simulink model "MultiRateCont"  (R2018b)
settings: Solver=ode4  StartTime=0.0  StopTime=10.0  FixedStep=.001  RelTol=1e-3
PreLoadFcn:
  | load 'test_data.mat'
values from neighbouring files (symbols this model uses):
  B = 234    [test_data.mat]
  B_inline = 3.14    [test_data.mat]
  C = 123    [test_data.mat]
libraries: simulink x1
settings Model: SimulationMode=rapid-accelerator  Creator=mmcbroom  LastModifiedBy=slentine
settings DataIOCC: LimitDataPoints=on  SignalLoggingSaveFormat=ModelDataLogs  SaveOutput=off  SignalLogging=off  DSMLogging=off  SaveTime=off
settings OptimizationCC: DefaultParameterBehavior=Inlined  EnhancedBackFolding=on  PassReuseOutputArgsAs=Individual arguments  ExpressionDepthLimit=2147483647  InitFltsAndDblsToZero=on  OptimizeBlockOrder=speed  DifferentSizesBufferReuse=on  OptimizationCustomize=off
settings DebuggingCC: SaveWithParameterizedLinksMsg=none  UnderspecifiedInitializationDetection=Classic  MergeDetectMultiDrivingBlocksExec=none  SolverPrmCheckMsg=warning  ParameterTunabilityLossMsg=error  FcnCallInpInsideContextMsg=warning  BusObjectLabelMismatch=none  StateNameClashWarn=warning  SFUnexpectedBacktrackingDiag=warning  SFNoUnconditionalDefaultTransitionDiag=warning  SFExecutionAtInitializationDiag=none
settings HardwareCC: ProdBitPerPointer=32  ProdBitPerSizeT=32  ProdBitPerPtrDiffT=32  ProdWordSize=32  ProdHWDeviceType=Intel->x86-32 (Windows32)
settings ModelReferenceCC: PropagateSignalLabelsOutOfModel=off
settings SFSimCC: SimUseLocalCustomCode=off  SimParseCustomCode=off  MATLABDynamicMemAlloc=off
settings RTWCC: SystemTargetFile=cfs_ert.tlc  TemplateMakefile=ert_default_tmf  Description=NASA CFS Target File  GenerateReport=on  RTWUseLocalCustomCode=off  IncludeHyperlinkInReport=on  LaunchReport=on  PortableWordSizes=on  GenerateTraceInfo=on  GenerateTraceReport=on  GenerateTraceReportSl=on  GenerateTraceReportSf=on  GenerateTraceReportEml=on
settings CodeAppCC: ForceParamTrailComments=on  IgnoreCustomStorageClasses=off  OperatorAnnotations=on  SimulinkDataObjDesc=on  SFDataObjDesc=on  CustomSymbolStrType=$N$R$M  CustomCommentsFcn=trick_comments.m  InsertBlockDesc=on  EnableCustomComments=on  InternalIdentifier=Classic
settings STFCustomTargetCC: MultiwordLength=256  GenerateSampleERTMain=on  CombineOutputUpdateFcns=on  ERTCustomFileBanners=on  MultiInstanceERTCode=on  CodeInterfacePackaging=Reusable function  SupportNonInlinedSFcns=off  RemoveResetFunc=on  MATLABClassNameForMDSCustomization=Simulink.SoftwareTarget.ERTCustomization  UseToolchainInfoCompliant=on  SystemTargetFile=cfs_ert.tlc
settings ERTTargetCC: GenerateSampleERTMain=on  ParMdlRefBuildCompliant=off  CompOptLevelCompliant=off  ConcurrentExecutionCompliant=off  MultiInstanceERTCode=on  CodeInterfacePackaging=Reusable function  SupportContinuousTime=on  ModelStepFunctionPrototypeControlCompliant=off  CPPClassGenCompliant=off  InlinedParameterPlacement=NonHierarchical  ERTCustomFileTemplate=cfs_interface.tlc
settings ConfigComp: CovMetricSettings=dw  CovHtmlReporting=on  CovSaveCumulativeToWorkspaceVar=on  CovSaveSingleToWorkspaceVar=on  CovExternalEMLEnable=off  CovSFcnEnable=off

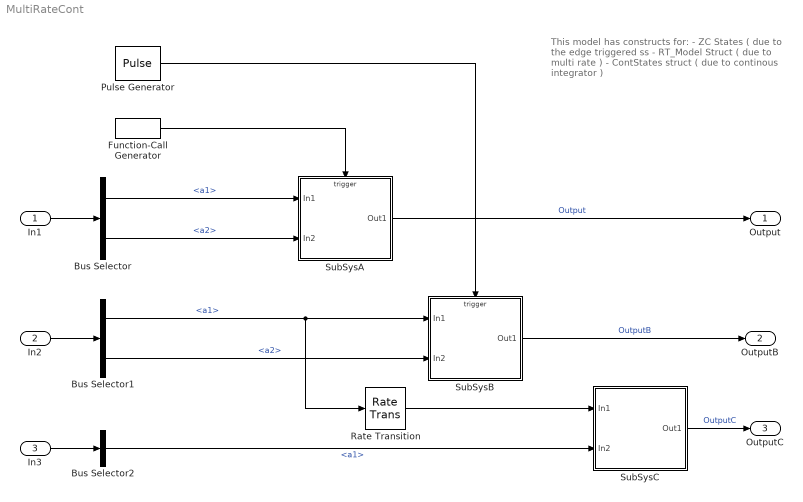
== system MultiRateCont ==
  note: This model has constructs for:
      | - ZC States ( due to the edge triggered ss
      | - RT_Model Struct ( due to multi rate )
      | - ContStates struct ( due to continous integrator )
  In1 : Inport  OutDataTypeStr=Bus: InBus_msg  BusOutputAsStruct=on
  In2 : Inport  Port=2  OutDataTypeStr=Bus: env_cmd_msg  BusOutputAsStruct=on
  In3 : Inport  Port=3  OutDataTypeStr=Bus: InBus_msg  SampleTime=.1  BusOutputAsStruct=on
  Bus Selector : BusSelector  OutputSignals=a1,a2
  Bus Selector1 : BusSelector  OutputSignals=a1,a2
  Bus Selector2 : BusSelector  OutputSignals=a1
  Function-Call Generator : simulink/Ports & Subsystems/Function-Call Generator  sample_time=1  numberOfIterations=1
  Pulse Generator : DiscretePulseGenerator  PulseType=Time based  PulseWidth=50
  Rate Transition : RateTransition  OutPortSampleTime=.1
  SubSysA : Subsystem
      settings: RTWFcnNameOpts=Use subsystem name
  SubSysB : Subsystem
      settings: RTWFcnNameOpts=Use subsystem name
  SubSysC : Subsystem
      settings: RTWSystemCode=Nonreusable function  RTWFcnNameOpts=Use subsystem name  RTWFileNameOpts=Use subsystem name
  Output : Outport
  OutputB : Outport  Port=2
  OutputC : Outport  Port=3
  wires:
  SubSysA/1(Out1) -> Output/1  "Output"
  SubSysB/1(Out1) -> OutputB/1  "OutputB"
  SubSysC/1(Out1) -> OutputC/1  "OutputC"
  Pulse Generator/1 -> SubSysB/Trigger
  Function-Call Generator/1 -> SubSysA/Trigger
  Rate Transition/1 -> SubSysC/1(In1)
  In1/1 -> Bus Selector/1
  Bus Selector/1 -> SubSysA/1(In1)  "<a1>"
  Bus Selector/2 -> SubSysA/2(In2)  "<a2>"
  In2/1 -> Bus Selector1/1
  Bus Selector1/1 -> SubSysB/1(In1), Rate Transition/1  "<a1>"
  Bus Selector1/2 -> SubSysB/2(In2)  "<a2>"
  In3/1 -> Bus Selector2/1
  Bus Selector2/1 -> SubSysC/2(In2)  "<a1>"

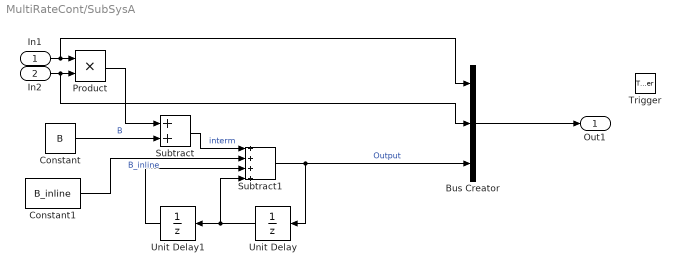
== system MultiRateCont/SubSysA ==
  In1 : Inport
  In2 : Inport  Port=2
  Trigger : TriggerPort  TriggerType=function-call  VariantControl=(inherit)
  Bus Creator : BusCreator  Inputs=3  OutDataTypeStr=Bus: OutBus_msg  NonVirtualBus=on
  Constant : Constant  Value=B
  Constant1 : Constant  Value=B_inline
  Product : Product  RndMeth=Zero
  Subtract : Sum
  Subtract1 : Sum  Inputs=++++
  Unit Delay : UnitDelay  SampleTime=-1  StateName=UnitDelayState
  Unit Delay1 : UnitDelay  SampleTime=-1
  Out1 : Outport
  wires:
  Product/1 -> Subtract/1
  Constant/1 -> Subtract/2  "B"
  Subtract/1 -> Subtract1/1  "interm"
  Subtract1/1 -> Unit Delay/1, Bus Creator/3  "Output"
  Constant1/1 -> Subtract1/2  "B_inline"
  Unit Delay/1 -> Subtract1/4, Unit Delay1/1
  Unit Delay1/1 -> Subtract1/3
  In1/1 -> Product/1, Bus Creator/1
  In2/1 -> Product/2, Bus Creator/2
  Bus Creator/1 -> Out1/1

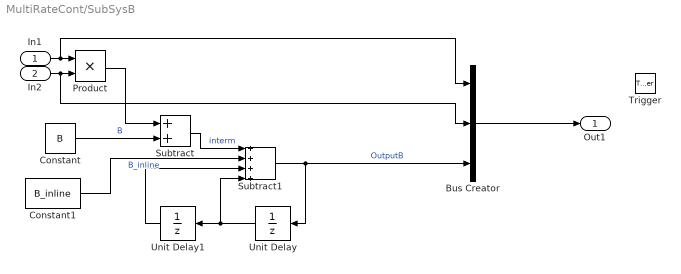
== system MultiRateCont/SubSysB ==
  In1 : Inport
  In2 : Inport  Port=2
  Trigger : TriggerPort  VariantControl=(inherit)
  Bus Creator : BusCreator  Inputs=3  OutDataTypeStr=Bus: gnc_cmd_msg  NonVirtualBus=on
  Constant : Constant  Value=B
  Constant1 : Constant  Value=B_inline
  Product : Product  RndMeth=Zero
  Subtract : Sum
  Subtract1 : Sum  Inputs=++++
  Unit Delay : UnitDelay  SampleTime=-1  StateName=UnitDelayState
  Unit Delay1 : UnitDelay  SampleTime=-1
  Out1 : Outport
  wires:
  Bus Creator/1 -> Out1/1
  In2/1 -> Bus Creator/2, Product/2
  In1/1 -> Bus Creator/1, Product/1
  Unit Delay1/1 -> Subtract1/3
  Unit Delay/1 -> Unit Delay1/1, Subtract1/4
  Constant1/1 -> Subtract1/2  "B_inline"
  Subtract1/1 -> Bus Creator/3, Unit Delay/1  "OutputB"
  Subtract/1 -> Subtract1/1  "interm"
  Constant/1 -> Subtract/2  "B"
  Product/1 -> Subtract/1

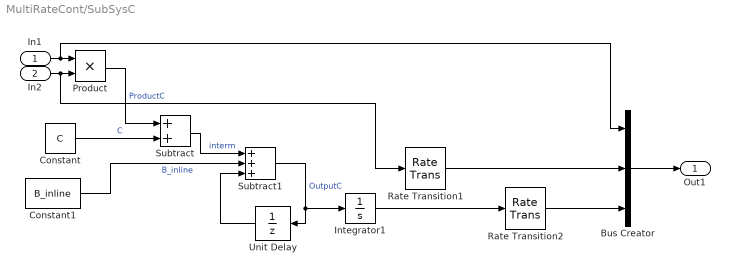
== system MultiRateCont/SubSysC ==
  In1 : Inport
  In2 : Inport  Port=2
  Bus Creator : BusCreator  Inputs=3  OutDataTypeStr=Bus: gnc_cmd_msg  NonVirtualBus=on
  Constant : Constant  Value=C
  Constant1 : Constant  Value=B_inline
  Integrator1 : Integrator
  Product : Product  RndMeth=Zero
  Rate Transition1 : RateTransition
  Rate Transition2 : RateTransition
  Subtract : Sum
  Subtract1 : Sum  Inputs=+++
  Unit Delay : UnitDelay  SampleTime=-1  StateName=UnitDelayStateC
  Out1 : Outport
  wires:
  In2/1 -> Product/2, Rate Transition1/1
  In1/1 -> Product/1, Bus Creator/1
  Subtract1/1 -> Unit Delay/1, Integrator1/1  "OutputC"
  Subtract/1 -> Subtract1/1  "interm"
  Constant/1 -> Subtract/2  "C"
  Product/1 -> Subtract/1  "ProductC"
  Constant1/1 -> Subtract1/2  "B_inline"
  Unit Delay/1 -> Subtract1/3
  Bus Creator/1 -> Out1/1
  Integrator1/1 -> Rate Transition2/1
  Rate Transition1/1 -> Bus Creator/2
  Rate Transition2/1 -> Bus Creator/3
